simulink library "sm_boom_lift_crawler_lib_actuators"  (R2026a)
settings: Solver=ode23t
undefined symbols (not defined in the file): actuators, BasketR, cylinders, Extend, Jib, LevelM, LevelS, Lift, lines, OutFL, OutFR, OutRL, OutRR, Tilt, TrackL, TrackR, Turret, valves
libraries: SimscapeFluids_lib x92, fl_lib x67, sm_boom_lift_crawler_lib x24, nesl_utility x13, Custom_Valves x2
(part 2 of 5)

== system sm_boom_lift_crawler_lib_actuators/Actuators/Hydraulic Power Unit/Diesel Pumps ==
  Ideal Angular Velocity Source : fl_lib/Mechanical/Mechanical Sources/Ideal Angular Velocity Source
  Mechanical Rotational Reference : fl_lib/Mechanical/Rotational Elements/Mechanical Rotational Reference
  Mechanical Rotational Reference1 : fl_lib/Mechanical/Rotational Elements/Mechanical Rotational Reference
  Mechanical Rotational Reference2 : fl_lib/Mechanical/Rotational Elements/Mechanical Rotational Reference
  Pump 1 : SimscapeFluids_lib/Isothermal Liquid/Pumps & Motors/Fixed-Displacement Pump (IL)  leakage_friction_spec=fluids.isothermal_liquid.pumps_motors.enum.pump_motor_loss_spec.analytical  displacement=6.67 cm^3/rev  omega_nominal=3500 rpm  p_nominal=3625 psi  vol_eff_nominal=0.97  mech_eff_nominal=0.6236256848969084  no_load_torque=9 in*lbf  p_diff_eff_TLU=[100000, 1000000, 2000000] Pa  omega_eff_TLU=[25, 50, 100, 200, 300, 400] rad/s  vol_eff_TLU=[.816, .908, .954, .977, .981, .984; .325, .663, .831, .916, .925, .946; .137, .568, .78, .892, .893, .91]  mech_eff_TLU=[.996, .996, .996, .996, .996, .996; .988, .989, .989, .989, .989, .99; .981, .981, .982, .982, .983, .984]  p_diff_loss_TLU=[100000, 1000000, 2000000] Pa  omega_loss_TLU=[25, 50, 100, 200, 300, 400] rad/s  vol_loss_TLU=[.023, .023, .023, .023, .0285, .032; .0844, .0842, .0845, .084, .1125, .108; .1079, .108, .11, .108, .1605, .18] * 1e-3 m^3/s  mech_loss_TLU=[.002, .002, .002, .002, .002, .002; .0607, .0556, .0556, .0556, .0556, .0505; .1937, .1937, .1833, .1833, .1729, .1626] N*m  vol_eff_min=1e-3  vol_eff_max=1  mech_eff_min=1e-3  mech_eff_max=1  pressure_threshold=1e5 Pa  omega_threshold=10 rad/s  supplied_range_check=simscape.enum.assert.action.none  pump_mode_check=simscape.enum.assert.action.none  pressure_check=simscape.enum.assert.action.none  p_min_valid=0 + 101325 Pa
  Pump 2 : SimscapeFluids_lib/Isothermal Liquid/Pumps & Motors/Fixed-Displacement Pump (IL)  leakage_friction_spec=fluids.isothermal_liquid.pumps_motors.enum.pump_motor_loss_spec.analytical  displacement=6.67 cm^3/rev  omega_nominal=3500 rpm  p_nominal=3625 psi  vol_eff_nominal=0.97  mech_eff_nominal=0.6236256848969084  no_load_torque=9 in*lbf  p_diff_eff_TLU=[100000, 1000000, 2000000] Pa  omega_eff_TLU=[25, 50, 100, 200, 300, 400] rad/s  vol_eff_TLU=[.816, .908, .954, .977, .981, .984; .325, .663, .831, .916, .925, .946; .137, .568, .78, .892, .893, .91]  mech_eff_TLU=[.996, .996, .996, .996, .996, .996; .988, .989, .989, .989, .989, .99; .981, .981, .982, .982, .983, .984]  p_diff_loss_TLU=[100000, 1000000, 2000000] Pa  omega_loss_TLU=[25, 50, 100, 200, 300, 400] rad/s  vol_loss_TLU=[.023, .023, .023, .023, .0285, .032; .0844, .0842, .0845, .084, .1125, .108; .1079, .108, .11, .108, .1605, .18] * 1e-3 m^3/s  mech_loss_TLU=[.002, .002, .002, .002, .002, .002; .0607, .0556, .0556, .0556, .0556, .0505; .1937, .1937, .1833, .1833, .1729, .1626] N*m  vol_eff_min=1e-3  vol_eff_max=1  mech_eff_min=1e-3  mech_eff_max=1  pressure_threshold=1e5 Pa  omega_threshold=10 rad/s  supplied_range_check=simscape.enum.assert.action.none  pump_mode_check=simscape.enum.assert.action.none  pressure_check=simscape.enum.assert.action.none  p_min_valid=0 + 101325 Pa
  Pump Speed : fl_lib/Physical Signals/Sources/PS Constant  constant=3200 rpm
      settings: AttributesFormatString=%<constant> %<constant_unit>
  P1 : PMIOPort  Side=Right
  P2 : PMIOPort  Port=2  Side=Right
  T1 : PMIOPort  Port=3  Side=Left
  T2 : PMIOPort  Port=4  Side=Left
  connections:
  Pump Speed/RConn1 -- Ideal Angular Velocity Source/RConn1
  Ideal Angular Velocity Source/RConn2 -- Mechanical Rotational Reference/LConn1
  Pump 1/RConn3 -- T1/RConn1
  Pump 2/RConn3 -- T2/RConn1
  P2/RConn1 -- Pump 2/LConn1
  Pump 2/RConn2 -- Mechanical Rotational Reference1/LConn1
  Ideal Angular Velocity Source/LConn1 -- Pump 2/RConn1 -- Pump 1/RConn1
  P1/RConn1 -- Pump 1/LConn1
  Pump 1/RConn2 -- Mechanical Rotational Reference2/LConn1

== system sm_boom_lift_crawler_lib_actuators/Actuators/Hydraulic Power Unit/Electrical Pumps ==
  Ideal Angular Velocity Source : fl_lib/Mechanical/Mechanical Sources/Ideal Angular Velocity Source
  Mechanical Rotational Reference1 : fl_lib/Mechanical/Rotational Elements/Mechanical Rotational Reference
  Mechanical Rotational Reference : fl_lib/Mechanical/Rotational Elements/Mechanical Rotational Reference
  Mechanical Rotational Reference2 : fl_lib/Mechanical/Rotational Elements/Mechanical Rotational Reference
  Pump 1 : SimscapeFluids_lib/Isothermal Liquid/Pumps & Motors/Fixed-Displacement Pump (IL)  leakage_friction_spec=fluids.isothermal_liquid.pumps_motors.enum.pump_motor_loss_spec.analytical  displacement=2.15 cm^3/rev  omega_nominal=4000 rpm  p_nominal=4600 psi  vol_eff_nominal=0.97  mech_eff_nominal=0.3512349596799828  no_load_torque=9 in*lbf  p_diff_eff_TLU=[100000, 1000000, 2000000] Pa  omega_eff_TLU=[25, 50, 100, 200, 300, 400] rad/s  vol_eff_TLU=[.816, .908, .954, .977, .981, .984; .325, .663, .831, .916, .925, .946; .137, .568, .78, .892, .893, .91]  mech_eff_TLU=[.996, .996, .996, .996, .996, .996; .988, .989, .989, .989, .989, .99; .981, .981, .982, .982, .983, .984]  p_diff_loss_TLU=[100000, 1000000, 2000000] Pa  omega_loss_TLU=[25, 50, 100, 200, 300, 400] rad/s  vol_loss_TLU=[.023, .023, .023, .023, .0285, .032; .0844, .0842, .0845, .084, .1125, .108; .1079, .108, .11, .108, .1605, .18] * 1e-3 m^3/s  mech_loss_TLU=[.002, .002, .002, .002, .002, .002; .0607, .0556, .0556, .0556, .0556, .0505; .1937, .1937, .1833, .1833, .1729, .1626] N*m  vol_eff_min=1e-3  vol_eff_max=1  mech_eff_min=1e-3  mech_eff_max=1  pressure_threshold=1e5 Pa  omega_threshold=10 rad/s  supplied_range_check=simscape.enum.assert.action.none  pump_mode_check=simscape.enum.assert.action.none  pressure_check=simscape.enum.assert.action.none  p_min_valid=0 + 101325 Pa
  Pump 2 : SimscapeFluids_lib/Isothermal Liquid/Pumps & Motors/Fixed-Displacement Pump (IL)  leakage_friction_spec=fluids.isothermal_liquid.pumps_motors.enum.pump_motor_loss_spec.analytical  displacement=2.15 cm^3/rev  omega_nominal=4000 rpm  p_nominal=4600 psi  vol_eff_nominal=0.97  mech_eff_nominal=0.3512349596799828  no_load_torque=9 in*lbf  p_diff_eff_TLU=[100000, 1000000, 2000000] Pa  omega_eff_TLU=[25, 50, 100, 200, 300, 400] rad/s  vol_eff_TLU=[.816, .908, .954, .977, .981, .984; .325, .663, .831, .916, .925, .946; .137, .568, .78, .892, .893, .91]  mech_eff_TLU=[.996, .996, .996, .996, .996, .996; .988, .989, .989, .989, .989, .99; .981, .981, .982, .982, .983, .984]  p_diff_loss_TLU=[100000, 1000000, 2000000] Pa  omega_loss_TLU=[25, 50, 100, 200, 300, 400] rad/s  vol_loss_TLU=[.023, .023, .023, .023, .0285, .032; .0844, .0842, .0845, .084, .1125, .108; .1079, .108, .11, .108, .1605, .18] * 1e-3 m^3/s  mech_loss_TLU=[.002, .002, .002, .002, .002, .002; .0607, .0556, .0556, .0556, .0556, .0505; .1937, .1937, .1833, .1833, .1729, .1626] N*m  vol_eff_min=1e-3  vol_eff_max=1  mech_eff_min=1e-3  mech_eff_max=1  pressure_threshold=1e5 Pa  omega_threshold=10 rad/s  supplied_range_check=simscape.enum.assert.action.none  pump_mode_check=simscape.enum.assert.action.none  pressure_check=simscape.enum.assert.action.none  p_min_valid=0 + 101325 Pa
  Pump Speed : fl_lib/Physical Signals/Sources/PS Constant  constant=1500 rpm
      settings: AttributesFormatString=%<constant> %<constant_unit>
  P1 : PMIOPort  Side=Left
  P2 : PMIOPort  Port=2  Side=Left
  T1 : PMIOPort  Port=3  Side=Right
  T2 : PMIOPort  Port=4  Side=Right
  connections:
  Ideal Angular Velocity Source/RConn1 -- Pump Speed/RConn1
  Mechanical Rotational Reference1/LConn1 -- Ideal Angular Velocity Source/RConn2
  Pump 1/RConn3 -- T1/RConn1
  Pump 2/RConn3 -- T2/RConn1
  P1/RConn1 -- Pump 1/LConn1
  Pump 1/RConn2 -- Mechanical Rotational Reference/LConn1
  P2/RConn1 -- Pump 2/LConn1
  Pump 2/RConn2 -- Mechanical Rotational Reference2/LConn1
  Ideal Angular Velocity Source/LConn1 -- Pump 2/RConn1 -- Pump 1/RConn1

== system sm_boom_lift_crawler_lib_actuators/Actuators/Sky Manifold/Bus Routing ==
  m1 : Inport
  m2 : Inport  Port=2
  Bus Creator : BusCreator  Inputs=8
  Bus Selector : BusSelector  OutputSignals=LevelS,LevelM,BasketR,Jib,Extend
  Bus Selector1 : BusSelector  OutputSignals=Turret,Lift,Tilt
  m : Outport
  wires:
  Bus Creator/1 -> m/1
  m1/1 -> Bus Selector/1
  m2/1 -> Bus Selector1/1
  Bus Selector1/1 -> Bus Creator/6  "<Turret>"
  Bus Selector1/2 -> Bus Creator/7  "<Lift>"
  Bus Selector1/3 -> Bus Creator/8  "<Tilt>"
  Bus Selector/1 -> Bus Creator/1  "<LevelS>"
  Bus Selector/2 -> Bus Creator/2  "<LevelM>"
  Bus Selector/3 -> Bus Creator/3  "<BasketR>"
  Bus Selector/4 -> Bus Creator/4  "<Jib>"
  Bus Selector/5 -> Bus Creator/5  "<Extend>"

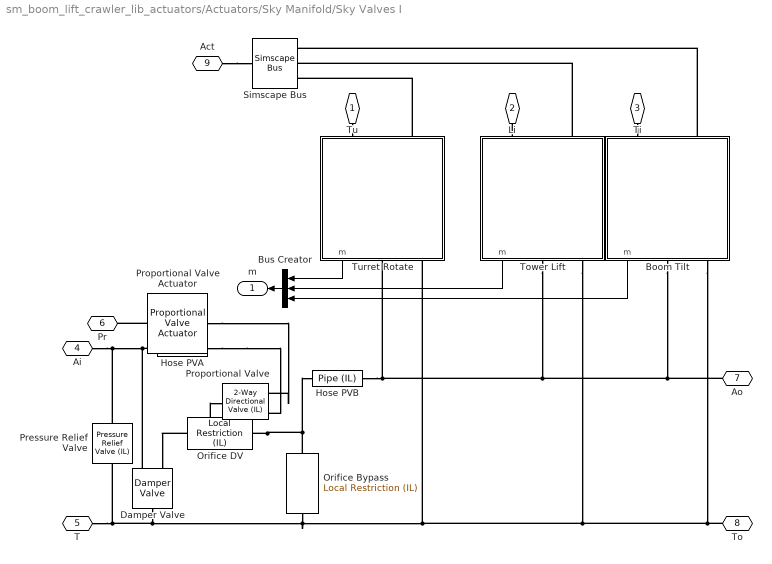
== system sm_boom_lift_crawler_lib_actuators/Actuators/Sky Manifold/Sky Valves I ==
  Boom Tilt : Subsystem
      mask Display: image('sh014.svg')
  Bus Creator : BusCreator  Inputs=3
  Damper Valve : Custom_Valves/Damper Valve  sMax=valves.control.l.max  T=2e-2  AMax=orifices.sky.d1.s  pCrack=25  pMax=75
  Hose PVA : SimscapeFluids_lib/Isothermal Liquid/Pipes & Fittings/Pipe (IL)  dynamic_compressibility=true  inertia=false  num_segments=1  pipe_length=lines.sky.main.l ft  cross_section_geometry=fluids.isothermal_liquid.pipes_fittings.enum.cross_section_geometry.circular  pipe_diameter=lines.sky.main.d.p in  pipe_inner_diameter=0.05 m  pipe_outer_diameter=0.1 m  pipe_width=0.1 m  pipe_height=0.1 m  pipe_major_axis=0.1 m  pipe_minor_axis=0.05 m  pipe_side=0.1 m  pipe_angle=30 deg  pipe_area=1e-4 m^2  Dh=1.12e-2 m  elevation_spec=foundation.enum.constant_variable.constant  elevation_gain=0 m  gravity_spec=foundation.enum.constant_variable.constant  g=9.81 m/s^2  pressure_loss_spec=fluids.isothermal_liquid.pipes_fittings.enum.pressure_loss_spec.haaland  mdot_nominal=[.1, 1] kg/s  p_diff_nominal=[.001, .01] MPa  mdot_threshold=1e-6 kg/s  local_pressure_loss_spec=fluids.isothermal_liquid.pipes_fittings.enum.local_loss_spec.aggregate_length  length_add=lines.sky.main.lr ft  loss_coefficient=0.1  roughness_spec=fluids.isothermal_liquid.pipes_fittings.enum.roughness_spec.custom  roughness=15e-6 m  Re_friction_TLU=[400, 1000, 1500, 3000, 4000, 6000, 10000, 20000, 40000, 60000, 100000, 100000000]  friction_factor_TLU=[.264, .112, .071, .0417, .0387, .0268, .025, .0232, .0226, .022, .0214, .0214]  Re_lam=2000  Re_tur=4000  shape_factor=64  pipe_wall_spec=fluids.isothermal_liquid.pipes_fittings.enum.wall_spec.rigid  vol_expansion_spec=fluids.isothermal_liquid.pipes_fittings.enum.vol_expansion_spec.area  area_pressure_gain=1e-6 m^2/MPa  static_pressure_TLU=[.1, 1] MPa  area_pressure_gain_TLU=[1e-05, 1.1e-05] m^2  material_behavior_spec=fluids.isothermal_liquid.pipes_fittings.enum.PipeMaterialBehavior.Linear  diameter_pressure_gain=2e-12 m/Pa  wall_thickness=0.05 m  elastic_modulus=69 GPa  stress_TLU=[276, 310] MPa  strain_TLU=[.004, .02]  stress_assert_action=simscape.enum.assert.action.none  stress_max=400 MPa  poisson_ratio=0.33  wall_time_constant=0.01 s  p0=lines.sky.main.p0 + 14.6959 psi  mdot0=0 kg/s
  Hose PVB : SimscapeFluids_lib/Isothermal Liquid/Pipes & Fittings/Pipe (IL)  dynamic_compressibility=true  inertia=false  num_segments=1  pipe_length=lines.sky.main.l ft  cross_section_geometry=fluids.isothermal_liquid.pipes_fittings.enum.cross_section_geometry.circular  pipe_diameter=lines.sky.main.d.p in  pipe_inner_diameter=0.05 m  pipe_outer_diameter=0.1 m  pipe_width=0.1 m  pipe_height=0.1 m  pipe_major_axis=0.1 m  pipe_minor_axis=0.05 m  pipe_side=0.1 m  pipe_angle=30 deg  pipe_area=1e-4 m^2  Dh=1.12e-2 m  elevation_spec=foundation.enum.constant_variable.constant  elevation_gain=0 m  gravity_spec=foundation.enum.constant_variable.constant  g=9.81 m/s^2  pressure_loss_spec=fluids.isothermal_liquid.pipes_fittings.enum.pressure_loss_spec.haaland  mdot_nominal=[.1, 1] kg/s  p_diff_nominal=[.001, .01] MPa  mdot_threshold=1e-6 kg/s  local_pressure_loss_spec=fluids.isothermal_liquid.pipes_fittings.enum.local_loss_spec.aggregate_length  length_add=lines.sky.main.lr ft  loss_coefficient=0.1  roughness_spec=fluids.isothermal_liquid.pipes_fittings.enum.roughness_spec.custom  roughness=15e-6 m  Re_friction_TLU=[400, 1000, 1500, 3000, 4000, 6000, 10000, 20000, 40000, 60000, 100000, 100000000]  friction_factor_TLU=[.264, .112, .071, .0417, .0387, .0268, .025, .0232, .0226, .022, .0214, .0214]  Re_lam=2000  Re_tur=4000  shape_factor=64  pipe_wall_spec=fluids.isothermal_liquid.pipes_fittings.enum.wall_spec.rigid  vol_expansion_spec=fluids.isothermal_liquid.pipes_fittings.enum.vol_expansion_spec.area  area_pressure_gain=1e-6 m^2/MPa  static_pressure_TLU=[.1, 1] MPa  area_pressure_gain_TLU=[1e-05, 1.1e-05] m^2  material_behavior_spec=fluids.isothermal_liquid.pipes_fittings.enum.PipeMaterialBehavior.Linear  diameter_pressure_gain=2e-12 m/Pa  wall_thickness=0.05 m  elastic_modulus=69 GPa  stress_TLU=[276, 310] MPa  strain_TLU=[.004, .02]  stress_assert_action=simscape.enum.assert.action.none  stress_max=400 MPa  poisson_ratio=0.33  wall_time_constant=0.01 s  p0=lines.sky.main.p0 + 14.6959 psi  mdot0=0 kg/s
  Orifice Bypass : fl_lib/Isothermal Liquid/Elements/Local Restriction (IL)  restriction_type=1  restriction_area=orifices.sky.d1.s in^2  min_area=1e-10 m^2  max_area=0.005 m^2  area=inf in^2  Cd=0.7  Re_c=150  pressure_recovery=simscape.enum.onoff.off
  Orifice DV : fl_lib/Isothermal Liquid/Elements/Local Restriction (IL)  restriction_type=1  restriction_area=orifices.sky.d1.s in^2  min_area=1e-10 m^2  max_area=0.005 m^2  area=inf in^2  Cd=0.7  Re_c=150  pressure_recovery=simscape.enum.onoff.off
  Pressure Relief Valve : SimscapeFluids_lib/Isothermal Liquid/Valves & Orifices/Pressure Control Valves/Pressure Relief Valve (IL)  set_pressure_spec=foundation.enum.constant_controlled.constant  opening_spec=1  pressure_spec=fluids.isothermal_liquid.valves_orifices.enum.pressure_control_spec.dp  p_set_gauge=0.1 MPa  p_set_differential=valves.relief.p.main psi  p_range=valves.relief.dp psi  area_max=lines.sky.main.s.p in^2  area_leak=1e-12 m^2  p_diff_TLU=[30.15e5 : 15e3 : 31.35e5] Pa  p_gauge_TLU=[0.2 : 0.2 : 1.2] MPa  valve_area_TLU=[1 : 1 : 9] .* 1e-5 m^2  vol_flow_TLU=[1e-09, 3.6e-05, 8.9e-05, .00015, .00023, .00031] m^3/s  area=inf m^2  Cd=0.7  Re_c=150  smoothing_factor=0.01  pressure_recovery=false  opening_dynamics=1  tau=2e-2 s
  Proportional Valve : SimscapeFluids_lib/Isothermal Liquid/Valves & Orifices/Directional Control Valves/2-Way Directional Valve (IL)  valve_spec=1  S_max=-(0) + (valves.control.l.max) in  del_S_max=0.00064516*(-(0) + (valves.control.l.max)) - ((valves.control.l.max)/(lines.sky.main.s.p)*(1e-12) - 0.00064516*(0)) m^2/in  area_max=lines.sky.main.s.p in^2  area_leak=1e-12 m^2  del_S_TLU="[0       0.002       0.004       0.007       0.017] m"  orifice_area_TLU=[1e-09, 2.0352e-07, 4.0736e-05, .00011438, .00034356] m^2  del_S_vol_flow_TLU="[0       0.002       0.004       0.007       0.017] m"  p_diff_TLU=[-10000000, -5000000, -2000000, 2000000, 5000000, 10000000] Pa  vol_flow_TLU=[-1e-07, -7.0711e-08, -4.4721e-08, 4.4721e-08, 7.0711e-08, 1e-07; -2.0352e-05, -1.4391e-05, -9.1017e-06, 9.1017e-06, 1.4391e-05, 2.0352e-05; -.0040736, -.0028805, -.0018218, .0018218, .0028805, .0040736; -.011438, -.0080879, -.0051152, .0051152, .0080879, .011438; -.034356, -.024293, -.015364, .015364, .024293, .034356] m^3/s  Cd=0.7  Re_c=150  smoothing_factor=0.001  pressure_recovery=false  area=inf m^2
  "Proportional Valve Actuator " : SimscapeFluids_lib/Valve Actuators/Proportional Valve Actuator  gain=1 in  time_constant=valves.control.tau.d s  valve_stroke=valves.control.l.max in
  Simscape Bus : SimscapeBus  HierarchyStrings=Tilt;Lift;Turret
  Tower Lift : Subsystem
      mask Display: image('sh014.svg')
  Turret Rotate : Subsystem
      mask Display: image('sh013.svg')
  Tu : PMIOPort  Side=Left
  Li : PMIOPort  Port=2  Side=Left
  Ti : PMIOPort  Port=3  Side=Left
  Ai : PMIOPort  Port=4  Side=Right
  T : PMIOPort  Port=5  Side=Right
  Pr : PMIOPort  Port=6  Side=Left
  Ao : PMIOPort  Port=7  Side=Right
  To : PMIOPort  Port=8  Side=Right
  Act : PMIOPort  Port=9  Side=Left
  m : Outport
  wires:
  Boom Tilt/1(m) -> Bus Creator/3
  Bus Creator/1 -> m/1
  Turret Rotate/1(m) -> Bus Creator/1
  Tower Lift/1(m) -> Bus Creator/2
  connections:
  Act/RConn1 -- Simscape Bus/RConn1
  Boom Tilt/LConn2 -- Simscape Bus/LConn1
  Tower Lift/LConn2 -- Simscape Bus/LConn2
  Turret Rotate/LConn2 -- Simscape Bus/LConn3
  Hose PVA/RConn1 -- Proportional Valve/LConn2
  Turret Rotate/RConn1 -- Ao/RConn1 -- Boom Tilt/RConn1 -- Tower Lift/RConn1 -- Hose PVB/RConn1
  Pressure Relief Valve/RConn1 -- T/RConn1 -- Damper Valve/RConn1 -- Orifice Bypass/RConn1 -- To/RConn1 -- Boom Tilt/RConn2 -- Tower Lift/RConn2 -- Turret Rotate/RConn2
  Hose PVA/LConn1 -- Ai/RConn1 -- Pressure Relief Valve/LConn1 -- Damper Valve/LConn1
  "Proportional Valve Actuator "/RConn1 -- Proportional Valve/LConn1
  Tu/RConn1 -- Turret Rotate/LConn1
  Tower Lift/LConn1 -- Li/RConn1
  Ti/RConn1 -- Boom Tilt/LConn1
  "Proportional Valve Actuator "/LConn1 -- Pr/RConn1
  Orifice Bypass/LConn1 -- Hose PVB/LConn1 -- Proportional Valve/RConn1 -- Orifice DV/LConn1
  Orifice DV/RConn1 -- Damper Valve/LConn2

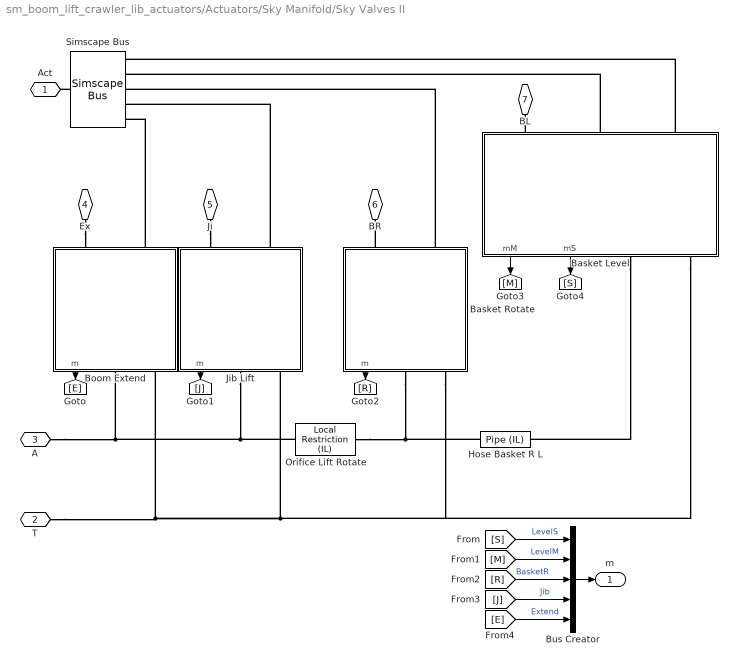
== system sm_boom_lift_crawler_lib_actuators/Actuators/Sky Manifold/Sky Valves II ==
  Basket Level : Subsystem
      mask Display: image('sh017.svg')
  Basket Rotate : Subsystem
      mask Display: image('sh016.svg')
  Boom Extend : Subsystem
      mask Display: image('sh015.svg')
  Bus Creator : BusCreator  Inputs=5
  Hose Basket R L : SimscapeFluids_lib/Isothermal Liquid/Pipes & Fittings/Pipe (IL)  dynamic_compressibility=true  inertia=false  num_segments=1  pipe_length=lines.sky.main.l ft  cross_section_geometry=fluids.isothermal_liquid.pipes_fittings.enum.cross_section_geometry.circular  pipe_diameter=lines.sky.main.d.p in  pipe_inner_diameter=0.05 m  pipe_outer_diameter=0.1 m  pipe_width=0.1 m  pipe_height=0.1 m  pipe_major_axis=0.1 m  pipe_minor_axis=0.05 m  pipe_side=0.1 m  pipe_angle=30 deg  pipe_area=1e-4 m^2  Dh=1.12e-2 m  elevation_spec=foundation.enum.constant_variable.constant  elevation_gain=0 m  gravity_spec=foundation.enum.constant_variable.constant  g=9.81 m/s^2  pressure_loss_spec=fluids.isothermal_liquid.pipes_fittings.enum.pressure_loss_spec.haaland  mdot_nominal=[.1, 1] kg/s  p_diff_nominal=[.001, .01] MPa  mdot_threshold=1e-6 kg/s  local_pressure_loss_spec=fluids.isothermal_liquid.pipes_fittings.enum.local_loss_spec.aggregate_length  length_add=lines.sky.main.lr ft  loss_coefficient=0.1  roughness_spec=fluids.isothermal_liquid.pipes_fittings.enum.roughness_spec.custom  roughness=15e-6 m  Re_friction_TLU=[400, 1000, 1500, 3000, 4000, 6000, 10000, 20000, 40000, 60000, 100000, 100000000]  friction_factor_TLU=[.264, .112, .071, .0417, .0387, .0268, .025, .0232, .0226, .022, .0214, .0214]  Re_lam=2000  Re_tur=4000  shape_factor=64  pipe_wall_spec=fluids.isothermal_liquid.pipes_fittings.enum.wall_spec.rigid  vol_expansion_spec=fluids.isothermal_liquid.pipes_fittings.enum.vol_expansion_spec.area  area_pressure_gain=1e-6 m^2/MPa  static_pressure_TLU=[.1, 1] MPa  area_pressure_gain_TLU=[1e-05, 1.1e-05] m^2  material_behavior_spec=fluids.isothermal_liquid.pipes_fittings.enum.PipeMaterialBehavior.Linear  diameter_pressure_gain=2e-12 m/Pa  wall_thickness=0.05 m  elastic_modulus=69 GPa  stress_TLU=[276, 310] MPa  strain_TLU=[.004, .02]  stress_assert_action=simscape.enum.assert.action.none  stress_max=400 MPa  poisson_ratio=0.33  wall_time_constant=0.01 s  p0=lines.sky.main.p0 + 14.6959 psi  mdot0=0 kg/s
  Jib Lift : Subsystem
      mask Display: image('sh014.svg')
  Orifice Lift Rotate : fl_lib/Isothermal Liquid/Elements/Local Restriction (IL)  restriction_type=1  restriction_area=orifices.sky.r2.s in^2  min_area=1e-10 m^2  max_area=0.005 m^2  area=inf in^2  Cd=0.7  Re_c=150  pressure_recovery=simscape.enum.onoff.off
  Simscape Bus : SimscapeBus  HierarchyStrings=LevelS;LevelM;BasketR;Jib;Extend
  Act : PMIOPort  Side=Left
  T : PMIOPort  Port=2  Side=Right
  A : PMIOPort  Port=3  Side=Right
  Ex : PMIOPort  Port=4  Side=Left
  Ji : PMIOPort  Port=5  Side=Left
  BR : PMIOPort  Port=6  Side=Left
  BL : PMIOPort  Port=7  Side=Left
  m : Outport
  wires:
  Basket Level/1(mM) -> [M]
  Basket Level/2(mS) -> [S]
  Boom Extend/1(m) -> [E]
  Jib Lift/1(m) -> [J]
  Basket Rotate/1(m) -> [R]
  [M] -> Bus Creator/2  "LevelM"
  [J] -> Bus Creator/4  "Jib"
  [R] -> Bus Creator/3  "BasketR"
  [E] -> Bus Creator/5  "Extend"
  [S] -> Bus Creator/1  "LevelS"
  Bus Creator/1 -> m/1
  connections:
  Basket Level/LConn3 -- Simscape Bus/LConn1
  Basket Level/LConn2 -- Simscape Bus/LConn2
  Basket Rotate/LConn2 -- Simscape Bus/LConn3
  Jib Lift/LConn2 -- Simscape Bus/LConn4
  Boom Extend/LConn2 -- Simscape Bus/LConn5
  Simscape Bus/RConn1 -- Act/RConn1
  Basket Rotate/RConn1 -- Orifice Lift Rotate/RConn1 -- Hose Basket R L/LConn1
  Ex/RConn1 -- Boom Extend/LConn1
  Ji/RConn1 -- Jib Lift/LConn1
  Basket Level/LConn1 -- BL/RConn1
  Basket Rotate/LConn1 -- BR/RConn1
  Basket Level/RConn1 -- Hose Basket R L/RConn1
  T/RConn1 -- Basket Rotate/RConn2 -- Basket Level/RConn2 -- Jib Lift/RConn2 -- Boom Extend/RConn2
  Jib Lift/RConn1 -- Orifice Lift Rotate/LConn1 -- Boom Extend/RConn1 -- A/RConn1

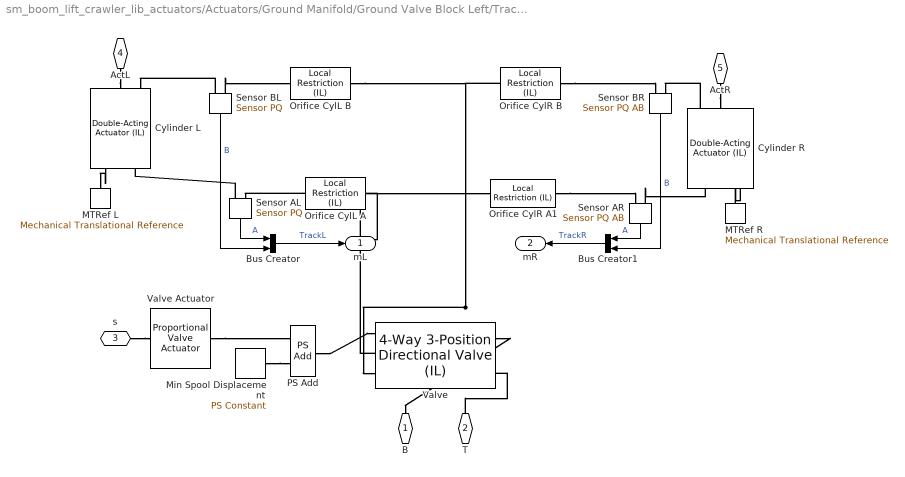
== system sm_boom_lift_crawler_lib_actuators/Actuators/Ground Manifold/Ground Valve Block Left/Track Extend ==
  " MTRef R" : fl_lib/Mechanical/Translational Elements/Mechanical Translational Reference
  Bus Creator : BusCreator  Inputs=2
  Bus Creator1 : BusCreator  Inputs=2
  Cylinder L : SimscapeFluids_lib/Isothermal Liquid/Actuators/Double-Acting Actuator (IL)  single_fluid=true  mech_orientation=1  piston_area_A=cylinders.ground.c5.s.a in^2  piston_area_B=cylinders.ground.c5.s.b in^2  stroke=cylinders.ground.c5.stroke in  dead_volume_A=cylinders.ground.c5.v.dead in^3  dead_volume_B=cylinders.ground.c5.v.dead in^3  pressure_spec=foundation.enum.pressure_spec.atmospheric  environment_pressure=0.101325 MPa  hardstop_model=simscape.enum.hardstop.smooth  stiff_coeff=cylinders.ground.c5.stops.kc N/m  damping_coeff=cylinders.ground.c5.stops.bc N/(m/s)  transition=1 mm  coeff_rest=0.2  v_tol=0.001 m/s  f_tol=0.001 N  cushion_A_spec=false  area_plunger_A=1e-4 m^2  length_plunger_A=1e-3 m  area_cushion_orifice_A=1e-6 m^2  area_leak_plunger_A=1e-7 m^2  p_crack_differential_A=0.01 MPa  press_max_differential_A=0.1 MPa  check_valve_area_max_A=1e-4 m^2  check_valve_area_leak_A=1e-10 m^2  smoothing_factor_A=0  cushion_B_spec=false  area_plunger_B=1e-4 m^2  length_plunger_B=1e-3 m  area_cushion_orifice_B=1e-6 m^2  area_leak_plunger_B=1e-7 m^2  p_crack_differential_B=0.01 MPa  press_max_differential_B=0.1 MPa  check_valve_area_max_B=1e-4 m^2  check_valve_area_leak_B=1e-10 m^2  smoothing_factor_B=0  friction_spec=false  breakaway_Coulomb_ratio=1.2  breakaway_velocity=0.1 m/s  preload_force=20 N  Coulomb_coeff=1e-6 N/Pa  viscous_coeff=100 N*s/m  leakage_spec=false  clearance=1e-4 m  piston_length=0.01 m  displacement_spec=foundation.enum.DisplacementSpec.Calculate  x0=0.01 in  dynamic_compressibility=true  p0_A=lines.ground.c5.p0.a + 14.6959 psi  p0_B=lines.ground.c5.p0.b + 14.6959 psi  p_nominal_A=0.101325 MPa  p_nominal_B=0.101325 MPa
      settings: LogSimulationData=on
  Cylinder R : SimscapeFluids_lib/Isothermal Liquid/Actuators/Double-Acting Actuator (IL)  single_fluid=true  mech_orientation=1  piston_area_A=cylinders.ground.c6.s.a in^2  piston_area_B=cylinders.ground.c6.s.b in^2  stroke=cylinders.ground.c6.stroke in  dead_volume_A=cylinders.ground.c6.v.dead in^3  dead_volume_B=cylinders.ground.c6.v.dead in^3  pressure_spec=foundation.enum.pressure_spec.atmospheric  environment_pressure=0.101325 MPa  hardstop_model=simscape.enum.hardstop.smooth  stiff_coeff=cylinders.ground.c6.stops.kc N/m  damping_coeff=cylinders.ground.c6.stops.bc N/(m/s)  transition=1 mm  coeff_rest=0.2  v_tol=0.001 m/s  f_tol=0.001 N  cushion_A_spec=false  area_plunger_A=1e-4 m^2  length_plunger_A=1e-3 m  area_cushion_orifice_A=1e-6 m^2  area_leak_plunger_A=1e-7 m^2  p_crack_differential_A=0.01 MPa  press_max_differential_A=0.1 MPa  check_valve_area_max_A=1e-4 m^2  check_valve_area_leak_A=1e-10 m^2  smoothing_factor_A=0  cushion_B_spec=false  area_plunger_B=1e-4 m^2  length_plunger_B=1e-3 m  area_cushion_orifice_B=1e-6 m^2  area_leak_plunger_B=1e-7 m^2  p_crack_differential_B=0.01 MPa  press_max_differential_B=0.1 MPa  check_valve_area_max_B=1e-4 m^2  check_valve_area_leak_B=1e-10 m^2  smoothing_factor_B=0  friction_spec=false  breakaway_Coulomb_ratio=1.2  breakaway_velocity=0.1 m/s  preload_force=20 N  Coulomb_coeff=1e-6 N/Pa  viscous_coeff=100 N*s/m  leakage_spec=false  clearance=1e-4 m  piston_length=0.01 m  displacement_spec=foundation.enum.DisplacementSpec.Calculate  x0=0.01 in  dynamic_compressibility=true  p0_A=lines.ground.c6.p0.a + 14.6959 psi  p0_B=lines.ground.c6.p0.b + 14.6959 psi  p_nominal_A=0.101325 MPa  p_nominal_B=0.101325 MPa
      settings: LogSimulationData=on
  MTRef L : fl_lib/Mechanical/Translational Elements/Mechanical Translational Reference
  Min Spool Displacement : fl_lib/Physical Signals/Sources/PS Constant  constant=1e-9 m
  Orifice CylL A : fl_lib/Isothermal Liquid/Elements/Local Restriction (IL)  restriction_type=1  restriction_area=1e-4 m^2  min_area=1e-10 m^2  max_area=0.005 m^2  area=inf m^2  Cd=0.7  Re_c=150  pressure_recovery=simscape.enum.onoff.off
  Orifice CylL B : fl_lib/Isothermal Liquid/Elements/Local Restriction (IL)  restriction_type=1  restriction_area=1e-4 m^2  min_area=1e-10 m^2  max_area=0.005 m^2  area=inf m^2  Cd=0.7  Re_c=150  pressure_recovery=simscape.enum.onoff.off
  Orifice CylR A1 : fl_lib/Isothermal Liquid/Elements/Local Restriction (IL)  restriction_type=1  restriction_area=1e-4 m^2  min_area=1e-10 m^2  max_area=0.005 m^2  area=inf m^2  Cd=0.7  Re_c=150  pressure_recovery=simscape.enum.onoff.off
  Orifice CylR B : fl_lib/Isothermal Liquid/Elements/Local Restriction (IL)  restriction_type=1  restriction_area=1e-4 m^2  min_area=1e-10 m^2  max_area=0.005 m^2  area=inf m^2  Cd=0.7  Re_c=150  pressure_recovery=simscape.enum.onoff.off
  PS Add : fl_lib/Physical Signals/Functions/PS Add
  Sensor AL : sm_boom_lift_crawler_lib/Sensor PQ  SystemSampleTime=-1  VariantActivationTime=update diagram  EmptyChoice=off  PassThrough=off  PassThroughVariantControl=(default)  EmptyChoiceVariantControl=(default)  AllowFlexibleInterface=on  Latency=0  AutoFrameSizeCalculation=off
  Sensor AR : sm_boom_lift_crawler_lib/Sensor PQ AB  SystemSampleTime=-1  VariantActivationTime=update diagram  EmptyChoice=off  PassThrough=off  PassThroughVariantControl=(default)  EmptyChoiceVariantControl=(default)  AllowFlexibleInterface=on  Latency=0  AutoFrameSizeCalculation=off
  Sensor BL : sm_boom_lift_crawler_lib/Sensor PQ  SystemSampleTime=-1  VariantActivationTime=update diagram  EmptyChoice=off  PassThrough=off  PassThroughVariantControl=(default)  EmptyChoiceVariantControl=(default)  AllowFlexibleInterface=on  Latency=0  AutoFrameSizeCalculation=off
  Sensor BR : sm_boom_lift_crawler_lib/Sensor PQ AB  SystemSampleTime=-1  VariantActivationTime=update diagram  EmptyChoice=off  PassThrough=off  PassThroughVariantControl=(default)  EmptyChoiceVariantControl=(default)  AllowFlexibleInterface=on  Latency=0  AutoFrameSizeCalculation=off
  Valve : SimscapeFluids_lib/Isothermal Liquid/Valves & Orifices/Directional Control Valves/4-Way 3-Position Directional Valve (IL)  open_orifices_pos=fluids.isothermal_liquid.valves_orifices.directional_control_valves.enum.directional_valve_open_orifices_pos_neg.PA_BT  open_orifices_neu=fluids.isothermal_liquid.valves_orifices.directional_control_valves.enum.directional_valve_open_orifices_neutral.all_closed  open_orifices_neg=fluids.isothermal_liquid.valves_orifices.directional_control_valves.enum.directional_valve_open_orifices_pos_neg.PB_AT  neutral_assert_action=0  area_spec=fluids.isothermal_liquid.valves_orifices.directional_control_valves.enum.directional_valve_area_spec.different  valve_spec=1  del_S_max=(valves.control.l.max) - (valves.control.l.max)/(lines.ground.c5.s)*(1e-9) in  area_max=lines.ground.c5.s in^2  del_S_TLU=[0, .00125, .0025, .00375, .005] m  valve_area_TLU=[1e-09, 2.0352e-07, 4.0736e-05, .00011438, .00034356] m^2  del_S_vol_flow_TLU=[0, .00125, .0025, .00375, .005] m  p_diff_TLU=[-10000000, -5000000, -2000000, 2000000, 5000000, 10000000] Pa  vol_flow_TLU=[-1e-07, -7.0711e-08, -4.4721e-08, 4.4721e-08, 7.0711e-08, 1e-07; -2.0352e-05, -1.4391e-05, -9.1017e-06, 9.1017e-06, 1.4391e-05, 2.0352e-05; -.0040736, -.0028805, -.0018218, .0018218, .0028805, .0040736; -.011438, -.0080879, -.0051152, .0051152, .0080879, .011438; -.034356, -.024293, -.015364, .015364, .024293, .034356] m^3/s  p_diff_TLU_const=[-.1, .3, .5, .7] MPa  vol_flow_TLU_const=[-.0009, .0016, .002, .0024] m^3/s  area_const=1e-4 m^2  area_leak=1e-9 in^2  area=inf m^2  Cd=0.7  Re_c=150  smoothing_factor=0.001  pressure_recovery=false  S_max_PA=-(0) + 0.0254*(valves.control.l.max) m  del_S_max_PA=(valves.control.l.max) - (valves.control.l.max)/(lines.ground.c5.s)*(1e-9) in  area_max_PA=lines.ground.c5.s in^2  del_S_TLU_PA=[0, .00125, .0025, .00375, .005] m  valve_area_TLU_PA=[1e-09, 2.0352e-07, 4.0736e-05, .00011438, .00034356] m^2  del_S_vol_flow_TLU_PA=[0, .00125, .0025, .00375, .005] m  p_diff_TLU_PA=[-10000000, -5000000, -2000000, 2000000, 5000000, 10000000] Pa  vol_flow_TLU_PA=[-1e-07, -7.0711e-08, -4.4721e-08, 4.4721e-08, 7.0711e-08, 1e-07; -2.0352e-05, -1.4391e-05, -9.1017e-06, 9.1017e-06, 1.4391e-05, 2.0352e-05; -.0040736, -.0028805, -.0018218, .0018218, .0028805, .0040736; -.011438, -.0080879, -.0051152, .0051152, .0080879, .011438; -.034356, -.024293, -.015364, .015364, .024293, .034356] m^3/s  area_const_PA=1e-4 m^2  p_diff_TLU_const_PA=[-.1, .3, .5, .7] MPa  vol_flow_TLU_const_PA=[-.0009, .0016, .002, .0024] m^3/s  S_max_PB=(0) - 0.0254*(valves.control.l.max) m  del_S_max_PB=(valves.control.l.max) - (valves.control.l.max)/(lines.ground.c5.s)*(1e-9) in  area_max_PB=lines.ground.c5.s in^2  del_S_TLU_PB=[0, .00125, .0025, .00375, .005] m  valve_area_TLU_PB=[1e-09, 2.0352e-07, 4.0736e-05, .00011438, .00034356] m^2  del_S_vol_flow_TLU_PB=[0, .00125, .0025, .00375, .005] m  p_diff_TLU_PB=[-10000000, -5000000, -2000000, 2000000, 5000000, 10000000] Pa  vol_flow_TLU_PB=[-1e-07, -7.0711e-08, -4.4721e-08, 4.4721e-08, 7.0711e-08, 1e-07; -2.0352e-05, -1.4391e-05, -9.1017e-06, 9.1017e-06, 1.4391e-05, 2.0352e-05; -.0040736, -.0028805, -.0018218, .0018218, .0028805, .0040736; -.011438, -.0080879, -.0051152, .0051152, .0080879, .011438; -.034356, -.024293, -.015364, .015364, .024293, .034356] m^3/s  area_const_PB=1e-4 m^2  p_diff_TLU_const_PB=[-.1, .3, .5, .7] MPa  vol_flow_TLU_const_PB=[-.0009, .0016, .002, .0024] m^3/s  S_max_AB=7.5e-3 m  del_S_max_AB=0.005 m  area_max_AB=1e-4 m^2  del_S_TLU_AB=[0, .00125, .0025, .00375, .005] m  valve_area_TLU_AB=[1e-10, 1e-05, 4e-05, 6e-05, .0001] m^2  del_S_vol_flow_TLU_AB=[0, .00125, .0025, .00375, .005] m  p_diff_TLU_AB=[-.1, .3, .5, .7] MPa  vol_flow_TLU_AB=[-1e-08, 2.2e-08, 2.8e-08, 3.4e-08; -9e-06, .00015, .0002, .00024; -.00036, .00063, .00081, .00096; -.00054, .00094, .0012, .0014; -.00091, .0016, .002, .0024] m^3/s  area_const_AB=1e-4 m^2  p_diff_TLU_const_AB=[-.1, .3, .5, .7] MPa  vol_flow_TLU_const_AB=[-.0009, .0016, .002, .0024] m^3/s  S_max_AT=(0) - 0.0254*(valves.control.l.max) m  del_S_max_AT=(valves.control.l.max) - (valves.control.l.max)/(lines.ground.main.s.t)*(1e-9) in  area_max_AT=lines.ground.main.s.t in^2  del_S_TLU_AT=[0, .00125, .0025, .00375, .005] m  valve_area_TLU_AT=[1e-09, 2.0352e-07, 4.0736e-05, .00011438, .00034356] m^2  del_S_vol_flow_TLU_AT=[0, .00125, .0025, .00375, .005] m  p_diff_TLU_AT=[-10000000, -5000000, -2000000, 2000000, 5000000, 10000000] Pa  vol_flow_TLU_AT=[-1e-07, -7.0711e-08, -4.4721e-08, 4.4721e-08, 7.0711e-08, 1e-07; -2.0352e-05, -1.4391e-05, -9.1017e-06, 9.1017e-06, 1.4391e-05, 2.0352e-05; -.0040736, -.0028805, -.0018218, .0018218, .0028805, .0040736; -.011438, -.0080879, -.0051152, .0051152, .0080879, .011438; -.034356, -.024293, -.015364, .015364, .024293, .034356] m^3/s  area_const_AT=1e-4 m^2  p_diff_TLU_const_AT=[-.1, .3, .5, .7] MPa  vol_flow_TLU_const_AT=[-.0009, .0016, .002, .0024] m^3/s  S_max_BT=-(0) + 0.0254*(valves.control.l.max) m  del_S_max_BT=(valves.control.l.max) - (valves.control.l.max)/(lines.ground.main.s.t)*(1e-9) in  area_max_BT=lines.ground.main.s.t in^2  del_S_TLU_BT=[0, .00125, .0025, .00375, .005] m  valve_area_TLU_BT=[1e-09, 2.0352e-07, 4.0736e-05, .00011438, .00034356] m^2  del_S_vol_flow_TLU_BT=[0, .00125, .0025, .00375, .005] m  p_diff_TLU_BT=[-10000000, -5000000, -2000000, 2000000, 5000000, 10000000] Pa  vol_flow_TLU_BT=[-1e-07, -7.0711e-08, -4.4721e-08, 4.4721e-08, 7.0711e-08, 1e-07; -2.0352e-05, -1.4391e-05, -9.1017e-06, 9.1017e-06, 1.4391e-05, 2.0352e-05; -.0040736, -.0028805, -.0018218, .0018218, .0028805, .0040736; -.011438, -.0080879, -.0051152, .0051152, .0080879, .011438; -.034356, -.024293, -.015364, .015364, .024293, .034356] m^3/s  area_const_BT=1e-4 m^2  p_diff_TLU_const_BT=[-.1, .3, .5, .7] MPa  vol_flow_TLU_const_BT=[-.0009, .0016, .002, .0024] m^3/s  S_max_PT=0 m  del_S_max_PT=0.005 m  area_max_PT=1e-4 m^2  del_S_TLU_PT=[0, .00125, .0025, .00375, .005] m  valve_area_TLU_PT=[1e-10, 1e-05, 4e-05, 6e-05, .0001] m^2  del_S_vol_flow_TLU_PT=[0, .00125, .0025, .00375, .005] m  p_diff_TLU_PT=[-.1, .3, .5, .7] MPa  vol_flow_TLU_PT=[-1e-08, 2.2e-08, 2.8e-08, 3.4e-08; -9e-06, .00015, .0002, .00024; -.00036, .00063, .00081, .00096; -.00054, .00094, .0012, .0014; -.00091, .0016, .002, .0024] m^3/s
  Valve Actuator : SimscapeFluids_lib/Valve Actuators/Proportional Valve Actuator  gain=1 in  time_constant=valves.control.tau.b s  valve_stroke=valves.control.l.max in
  B : PMIOPort  Side=Left
  T : PMIOPort  Port=2  Side=Left
  s : PMIOPort  Port=3  Side=Right
  ActL : PMIOPort  Port=4  Side=Right
  ActR : PMIOPort  Port=5  Side=Right
  mL : Outport
  mR : Outport  Port=2
  wires:
  Sensor BL/1 -> Bus Creator/2  "B"
  Sensor AL/1 -> Bus Creator/1  "A"
  Bus Creator/1 -> mL/1  "TrackL"
  Bus Creator1/1 -> mR/1  "TrackR"
  Sensor AR/1 -> Bus Creator1/1  "A"
  Sensor BR/1 -> Bus Creator1/2  "B"
  connections:
  Valve Actuator/RConn1 -- PS Add/LConn1
  Min Spool Displacement/RConn1 -- PS Add/LConn2
  s/RConn1 -- Valve Actuator/LConn1
  ActL/RConn1 -- Cylinder L/RConn2
  Sensor BL/LConn1 -- Cylinder L/RConn3
  Sensor AL/LConn1 -- Cylinder L/LConn2
  Cylinder L/LConn1 -- MTRef L/LConn1
  ActR/RConn1 -- Cylinder R/RConn2
  Cylinder R/RConn3 -- Sensor BR/LConn2
  Sensor AR/LConn2 -- Cylinder R/LConn2
  " MTRef R"/LConn1 -- Cylinder R/LConn1
  Orifice CylL A/RConn1 -- Sensor AL/LConn2
  Sensor BL/LConn2 -- Orifice CylL B/RConn1
  Orifice CylR A1/RConn1 -- Sensor AR/LConn1
  Orifice CylR B/RConn1 -- Sensor BR/LConn1
  Valve/LConn2 -- Orifice CylR A1/LConn1 -- Orifice CylL A/LConn1
  Valve/LConn3 -- Orifice CylL B/LConn1 -- Orifice CylR B/LConn1
  PS Add/RConn1 -- Valve/LConn1
  Valve/RConn1 -- B/RConn1
  T/RConn1 -- Valve/RConn2
